simulink model "CruishKontrol"  (R2021a)
settings: Solver=VariableStepAuto  StartTime=0.0  StopTime=10.0  RelTol=1e-3
settings Model: Creator=asus  LastModifiedBy=asus

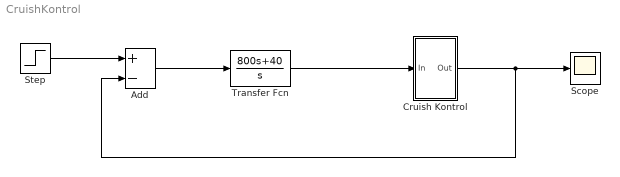
== system CruishKontrol ==
  Add : Sum  Inputs=+-
  Cruish Kontrol : Subsystem
  Scope : Scope
  Step : Step  SampleTime=0
  Transfer Fcn : TransferFcn  Numerator=[800 40]  Denominator=[1 0]
  wires:
  Step/1 -> Add/1
  Cruish Kontrol/1(Out) -> Add/2, Scope/1
  Transfer Fcn/1 -> Cruish Kontrol/1(In)
  Add/1 -> Transfer Fcn/1

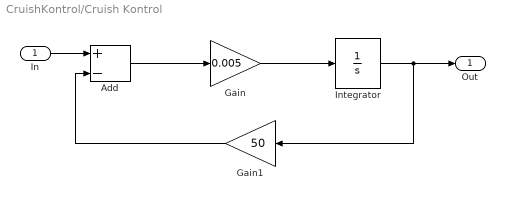
== system CruishKontrol/Cruish Kontrol ==
  In : Inport
  Add : Sum  Inputs=+-
  Gain : Gain  Gain=0.005
  Gain1 : Gain  Gain=50
  Integrator : Integrator
  Out : Outport
  wires:
  Integrator/1 -> Out/1, Gain1/1
  Add/1 -> Gain/1
  Gain1/1 -> Add/2
  Gain/1 -> Integrator/1
  In/1 -> Add/1
